simulink model "model3_cm"  (R2018b)
settings: Solver=FixedStepDiscrete  StartTime=0.0  StopTime=Inf  FixedStep=0.015  RelTol=1e-3  EnableMultiTasking=on
undefined symbols (not defined in the file): acA2000, Ace, Basler, FreeRun, PoCL, USETHISONE
libraries: dotFinder_ul x1, xpcbitflowlib x1, slrtlib x1, rayTrace_ul x1
settings Model: sg_rtwmakecfg_data=_bitflow_  SimulationMode=external  Creator=mcobb  LastModifiedBy=mae-ncsucore
settings SolverCC: ConcurrentTasks=on  AutoInsertRateTranBlk=on
settings DataIOCC: SaveFormat=StructureWithTime
settings OptimizationCC: BlockReduction=off  OptimizeBlockIOStorage=off  BufferReuse=off  GlobalBufferReuse=off  ExpressionFolding=off  LocalBlockOutputs=off  OptimizeDataStoreBuffers=off  BusAssignmentInplaceUpdate=off
settings DebuggingCC: LibraryContextMissingDiagnostic=none
settings HardwareCC: ProdBitPerPointer=32  ProdBitPerSizeT=32  ProdBitPerPtrDiffT=32  ProdLargestAtomicFloat=None  ProdWordSize=32  ProdLongLongMode=on  ProdHWDeviceType=Generic->32-bit x86 compatible
settings SFSimCC: SimUseLocalCustomCode=off
settings RTWCC: SystemTargetFile=slrt.tlc  TemplateMakefile=slrt_default_tmf  Description=Simulink Real-Time  RTWUseLocalCustomCode=off  CodeExecutionProfiling=on  RTWCompilerOptimization=on
settings SimulinkRealTimeCC: SupportVariableSizeSignals=on  PreserveStateflowLocalDataDimensions=off  RL32ObjectName=tg3  xPCisDefaultEnv=off  xPCTargetPCEnvName=Machine3  xPCConcurrentTasks=on

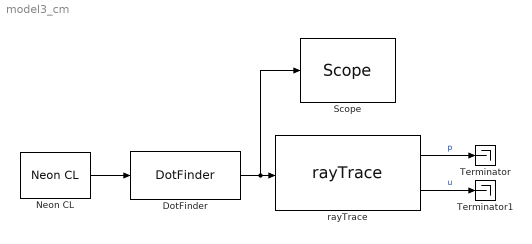
== system model3_cm ==
  DotFinder : dotFinder_ul/DotFinder  ROIPositionHoldEnable=off  ROIPositionHoldCoordinates=[650 1250]  ROIDimVec_px=[40 100]  ImageDimensions=[1000 2000]
  "Neon CL " : xpcbitflowlib/Neon CL   camerapath=Basler-Ace-acA2000-340km-E2-PoCL-FreeRun-USETHISONE.r64  r64=CAMERA  sampletime=0.015  slot=-1  make=Basler  model=acA2000-340km  mode=8 bit, 2 tap, 2048x1088, Free Run  owner=BitFlow  revision=1  modelcomp=0  revcomp=0  aqtimeout=4096  format=1  flashmux=Mux_2TOEP  flashdcc=DCC  pixbitdepth=8  xsize=2048  ysize=1088  xstart=0  ystart=0  dx=2048  dy=1088  expmod="[1  0]"  config="[4294967295         128;4294967295           0;4294967295           0;4294967295           0;4294967295           0;4294967295           0;4294967295      262144;4294967295           0;4294967295           0;4294967295           0;4294967295        1024;4294967295           0;4294967295           0;4294967295  4294967295;4294967295           0;4294967295           0;4294967295           0;4294967295      737280;4294967295        1088;4294967295           0;4294967295           0;4294967295           0;4294967295           0;4294967295           0;4294967295           0;4294967295           0;4294967295        7372;4294967295           0]"  ctab="[4      0     16      1   4112      2     16  32768      0]"  qtabmodel="[1   2048  65536]"  trigmode=0  baud=1  bytewidth=4  parity=1  stopbits=1  command="\"\""  response=0  comments=|
      | Free Run Mode / CC Trigger Mode
      | 
      | CC Trigger can be adjusted via GPV0 in CTAB
      | 
      | To use CC Trigger, camera must set to CC Trigger Mode.
      settings: SourceProductName=Simulink Real-Time: Speedgoat I/O Driver Library
  "Scope " : slrtlib/Displays and Logging/Scope   scopeno=1  scopetype=Target  autostart=on  viewmode=Numerical  formatstr='%15.6f'  grid=on  ylimits=[0,0]  nosamples=250  noprepostsamples=0  interleave=1  triggermode=FreeRun  triggersignal=1  trigsignalfromport=off  triggerlevel=0.0  triggerslope=Either  triggerscope=1  triggersample=0  filename=data.dat  mode=Lazy  writesize=512  autorestart=off  dynamicfilemode=off  maxwritefilesize=512*1024^2
  Terminator : Terminator
  Terminator1 : Terminator
  rayTrace : rayTrace_ul/rayTrace  camPosVec_cm=[1 1 1]  camEulAngles_deg=[0 0 0]  dist2Glass_cm=0  indOfRefVec=[0 0 0]  glassPlane=0  glassThickness_cm=0  imageDimsVec_px=[1000 2000]  camFOV_deg=[20 20]  Periscope=1
  wires:
  "Neon CL "/1 -> DotFinder/1
  DotFinder/1 -> "Scope "/1, rayTrace/1
  rayTrace/1 -> Terminator/1  "p"
  rayTrace/2 -> Terminator1/1  "u"
